simulink model "ClosedLoop_sim"  (Simulink 9.2)
settings: Solver=VariableStepAuto  StartTime=0.0  StopTime=10.0  RelTol=1e-3
libraries: neural x305, simulink x1
(part 1 of 13)
settings Model: Creator=manzand  LastModifiedBy=manzand
settings DataIOCC: LimitDataPoints=off  SaveFormat=Dataset  SignalLoggingSaveFormat=Dataset
settings OptimizationCC: LifeSpan=auto
settings DebuggingCC: UnderspecifiedInitializationDetection=Simplified  MergeDetectMultiDrivingBlocksExec=error  FcnCallInpInsideContextMsg=error  StateNameClashWarn=none  SFUnexpectedBacktrackingDiag=error  SFNoUnconditionalDefaultTransitionDiag=error  SFExecutionAtInitializationDiag=warning
settings HardwareCC: ProdBitPerPointer=64  ProdBitPerSizeT=64  ProdBitPerPtrDiffT=64  ProdLargestAtomicFloat=Float  ProdIntDivRoundTo=Zero  ProdEndianess=LittleEndian  ProdWordSize=64  ProdHWDeviceType=Intel->x86-64 (Windows64)
settings ModelReferenceCC: PropagateSignalLabelsOutOfModel=on
settings SFSimCC: SimUseLocalCustomCode=on
settings RTWCC: RTWUseLocalCustomCode=on
settings CodeAppCC: StateflowObjectComments=off
settings GRTTargetCC: TargetLangStandard=C99 (ISO)  GeneratePreprocessorConditionals=Use local settings  CombineOutputUpdateFcns=on  GRTInterface=off
settings ConfigComp: CovMetricSettings=dwe  CovHtmlReporting=off  CovSaveCumulativeToWorkspaceVar=off  CovSaveSingleToWorkspaceVar=off  CovExternalEMLEnable=on

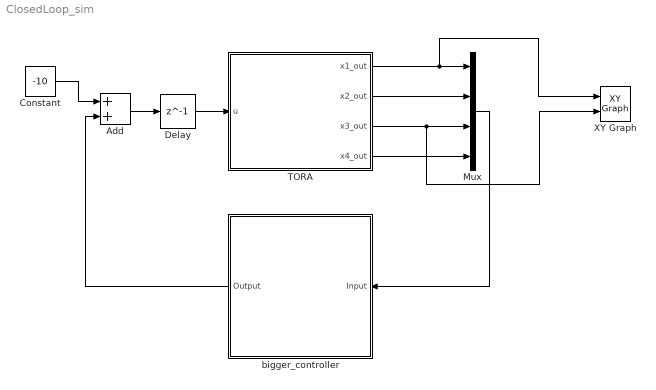
== system ClosedLoop_sim ==
  Add : Sum
  Constant : Constant  Value=-10
  Delay : Delay  DelayLength=1  InitialCondition=0
  Mux : Mux
  TORA : Stateflow chart  TreatAsAtomicUnit=on
  XY Graph : simulink/Sinks/XY Graph  xmin=-1  xmax=1  ymin=-1  ymax=1  st=-1
  bigger_controller : Subsystem
      mask help: Feed-Forward Neural Network
      mask Display: e = 0.06;c1 = [120 150 230]/255;c2 = ([120 150 230]+0)/383;c3 = ([120 150 230]+128)/383;patch([0 1 1 0],[0 0 1 1],c1);patch([0 1 1 1-e 1-e 0+e],[0 0 1 1-e 0+e 0+e],c2);patch([0 0 1 1-e 0+e 0+e],[0 1 1 1-e 1-e 0+e],c3);plot([0 1 1 0 0],[0 0 1 1 0]);fprintf('NNET');port_label('input',1,' Input');port_label('output',1,'Output ');
  wires:
  TORA/1(x1_out) -> XY Graph/1, Mux/1
  TORA/2(x2_out) -> Mux/2
  TORA/3(x3_out) -> XY Graph/2, Mux/3
  TORA/4(x4_out) -> Mux/4
  Add/1 -> Delay/1
  Constant/1 -> Add/1
  Mux/1 -> bigger_controller/1(Input)
  bigger_controller/1(Output) -> Add/2
  Delay/1 -> TORA/1(u)

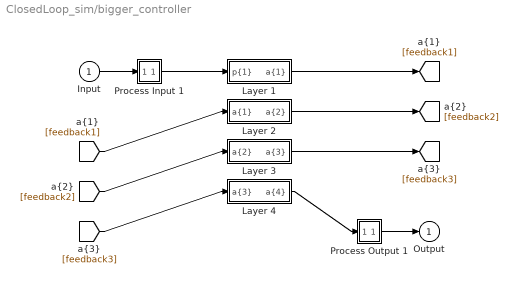
== system ClosedLoop_sim/bigger_controller ==
  Input : Inport  PortDimensions=4
      mask Display: e = 0.06;c1 = [120 230 180]/255;c2 = ([120 230 180]+0)/(256+128);c3 = ([120 230 180]+128)/(256+128);patch([0 1 1 0],[0 0 1 1],c1);patch([0 1 1 1-e 1-e 0+e],[0 0 1 1-e 0+e 0+e],c2);patch([0 0 1 1-e 0+e 0+e],[0 1 1 1-e 1-e 0+e],c3);plot([0 1 1 0 0],[0 0 1 1 0]);
  Layer 1 : Subsystem
      mask Display: e = 0.06;c1 = [120 150 230]/255;c2 = ([120 150 230]+0)/383;c3 = ([120 150 230]+128)/383;patch([0 1 1 0],[0 0 1 1],c1);patch([0 1 1 1-e 1-e 0+e],[0 0 1 1-e 0+e 0+e],c2);patch([0 0 1 1-e 0+e 0+e],[0 1 1 1-e 1-e 0+e],c3);plot([0 1 1 0 0],[0 0 1 1 0]);
  Layer 2 : Subsystem
      mask Display: e = 0.06;c1 = [120 150 230]/255;c2 = ([120 150 230]+0)/383;c3 = ([120 150 230]+128)/383;patch([0 1 1 0],[0 0 1 1],c1);patch([0 1 1 1-e 1-e 0+e],[0 0 1 1-e 0+e 0+e],c2);patch([0 0 1 1-e 0+e 0+e],[0 1 1 1-e 1-e 0+e],c3);plot([0 1 1 0 0],[0 0 1 1 0]);
  Layer 3 : Subsystem
      mask Display: e = 0.06;c1 = [120 150 230]/255;c2 = ([120 150 230]+0)/383;c3 = ([120 150 230]+128)/383;patch([0 1 1 0],[0 0 1 1],c1);patch([0 1 1 1-e 1-e 0+e],[0 0 1 1-e 0+e 0+e],c2);patch([0 0 1 1-e 0+e 0+e],[0 1 1 1-e 1-e 0+e],c3);plot([0 1 1 0 0],[0 0 1 1 0]);
  Layer 4 : Subsystem
      mask Display: e = 0.06;c1 = [120 150 230]/255;c2 = ([120 150 230]+0)/383;c3 = ([120 150 230]+128)/383;patch([0 1 1 0],[0 0 1 1],c1);patch([0 1 1 1-e 1-e 0+e],[0 0 1 1-e 0+e 0+e],c2);patch([0 0 1 1-e 0+e 0+e],[0 1 1 1-e 1-e 0+e],c3);plot([0 1 1 0 0],[0 0 1 1 0]);
  Process Input 1 : Subsystem
      mask Display: e = 0.06;c1 = [120 150 230]/255;c2 = ([120 150 230]+0)/383;c3 = ([120 150 230]+128)/383;patch([0 1 1 0],[0 0 1 1],c1);patch([0 1 1 1-e 1-e 0+e],[0 0 1 1-e 0+e 0+e],c2);patch([0 0 1 1-e 0+e 0+e],[0 1 1 1-e 1-e 0+e],c3);plot([0 1 1 0 0],[0 0 1 1 0]);
  Process Output 1 : Subsystem
      mask Display: e = 0.06;c1 = [120 150 230]/255;c2 = ([120 150 230]+0)/383;c3 = ([120 150 230]+128)/383;patch([0 1 1 0],[0 0 1 1],c1);patch([0 1 1 1-e 1-e 0+e],[0 0 1 1-e 0+e 0+e],c2);patch([0 0 1 1-e 0+e 0+e],[0 1 1 1-e 1-e 0+e],c3);plot([0 1 1 0 0],[0 0 1 1 0]);
  Output : Outport  InitialOutput=0
      mask Display: e = 0.06;c1 = [120 230 180]/255;c2 = ([120 230 180]+0)/(256+128);c3 = ([120 230 180]+128)/(256+128);patch([0 1 1 0],[0 0 1 1],c1);patch([0 1 1 1-e 1-e 0+e],[0 0 1 1-e 0+e 0+e],c2);patch([0 0 1 1-e 0+e 0+e],[0 1 1 1-e 1-e 0+e],c3);plot([0 1 1 0 0],[0 0 1 1 0]);
  wires:
  Layer 4/1("a{4}") -> Process Output 1/1(a)
  [feedback3] -> Layer 4/1("a{3} ")
  Layer 3/1("a{3}") -> [feedback3]
  [feedback2] -> Layer 3/1("a{2} ")
  Layer 2/1("a{2}") -> [feedback2]
  [feedback1] -> Layer 2/1("a{1} ")
  Layer 1/1("a{1}") -> [feedback1]
  Process Input 1/1(p) -> Layer 1/1("p{1}")
  Process Output 1/1(y) -> Output/1
  Input/1 -> Process Input 1/1(x)

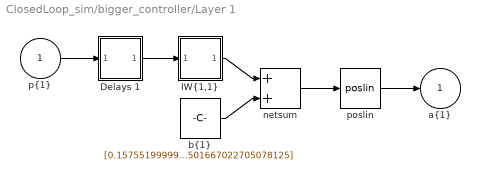
== system ClosedLoop_sim/bigger_controller/Layer 1 ==
  "p{1}" : Inport  PortDimensions=4
      mask Display: e = 0.06;c1 = [120 230 180]/255;c2 = ([120 230 180]+0)/(256+128);c3 = ([120 230 180]+128)/(256+128);patch([0 1 1 0],[0 0 1 1],c1);patch([0 1 1 1-e 1-e 0+e],[0 0 1 1-e 0+e 0+e],c2);patch([0 0 1 1-e 0+e 0+e],[0 1 1 1-e 1-e 0+e],c3);plot([0 1 1 0 0],[0 0 1 1 0]);
  Delays 1 : Subsystem
      mask Display: e = 0.06;c1 = [120 150 230]/255;c2 = ([120 150 230]+0)/383;c3 = ([120 150 230]+128)/383;patch([0 1 1 0],[0 0 1 1],c1);patch([0 1 1 1-e 1-e 0+e],[0 0 1 1-e 0+e 0+e],c2);patch([0 0 1 1-e 0+e 0+e],[0 1 1 1-e 1-e 0+e],c3);plot([0 1 1 0 0],[0 0 1 1 0]);disp('0');
  "IW{1,1}" : Subsystem
      mask Display: e = 0.06;c1 = [120 150 230]/255;c2 = ([120 150 230]+0)/383;c3 = ([120 150 230]+128)/383;patch([0 1 1 0],[0 0 1 1],c1);patch([0 1 1 1-e 1-e 0+e],[0 0 1 1-e 0+e 0+e],c2);patch([0 0 1 1-e 0+e 0+e],[0 1 1 1-e 1-e 0+e],c3);plot([0 1 1 0 0],[0 0 1 1 0]);disp('W');
  "b{1}" : Constant  Value=[0.1575519999999999976036946236490621231496334075927734375;0.17304500000000000436983782492461614310741424560546875;0.2687180000000000124060761663713492453098297119140625;0.179725999999999996870059248976758681237697601318359375;0.040231999999999996930899470726217259652912616729736328125;0.156368000000000006988187806200585328042507171630859375;0.31267699999999998272670609367196448147296905517578125;0.2392579999999999984527931928823818452656269073486328125;0.1582800000000000040234482412415673024952411651611328125;0.2311739999999999906066250332514755427837371826171875;0.2380319999999999935891281666044960729777812957763671875;0.246018999999999987693399816635064780712127685546875;0.236512000000000000010658141036401502788066864013671875;0.2016340000000000076685324756908812560141086578369140625;0.209523999999999988030907616121112369000911712646484375;0.299843000000000026172841671723290346562862396240234375;0.130168000000000005922373702560435049235820770263671875;0.1506659999999999943742778896194067783653736114501953125;0.1991340000000000054480864264405681751668453216552734375;0.189705000000000012505552149377763271331787109375;0.2312309999999999921005411351870861835777759552001953125;0.2230020000000000057749360848902142606675624847412109375;0.23258400000000001295319407290662638843059539794921875;0.107484999999999997211119762141606770455837249755859375;0.253188000000000024147794874807004816830158233642578125;0.20484700000000000130739863379858434200286865234375;0.2490779999999999938520289788357331417500972747802734375;0.32403199999999998670574541392852552235126495361328125;0.1958930000000000115623066676562302745878696441650390625;0.30651200000000000667199628878734074532985687255859375;0.1592550000000000076649797620120807550847530364990234375;0.20692399999999999682387397115235216915607452392578125;0.1734940000000000093205443363331141881644725799560546875;0.2635899999999999909761072558467276394367218017578125;0.201423999999999991938892662801663391292095184326171875;0.2122179999999999899795710689431871287524700164794921875;0.062077000000000000234923192010683123953640460968017578125;0.1976620000000000043627323975670151412487030029296875;0.10692300000000000415045775525868521071970462799072265625;0.22057599999999999429434183184639550745487213134765625;0.211060999999999998610888951589004136621952056884765625;0.165831000000000006178169087434071116149425506591796875;0.2300419999999999964845898148269043304026126861572265625;0.2126230000000000064375171859865076839923858642578125;0.22377700000000000368771679859491996467113494873046875;0.2484480000000000021742607714259065687656402587890625;0.1790090000000000014512835377900046296417713165283203125;0.300943000000000016047607687141862697899341583251953125;0.22207399999999999362643166023190133273601531982421875;0.1654730000000000089688256821318645961582660675048828125;0.3032880000000000020321522242738865315914154052734375;0.1556530000000000135695898961785132996737957000732421875;0.1670599999999999862865251998300664126873016357421875;0.227673999999999987498000564301037229597568511962890625;0.176128000000000006775024985472555272281169891357421875;0.2231769999999999865014643773974967189133167266845703125;0.279793000000000013915979479861562140285968780517578125;0.23367999999999999882760448599583469331264495849609375;0.164144000000000012118306358388508670032024383544921875;0.228663000000000005140776693224324844777584075927734375;0.1560140000000000137792000032277428545057773590087890625;0.195535999999999987597476547307451255619525909423828125;0.1807410000000000127595711774119990877807140350341796875;0.16601399999999999490540858460008166730403900146484375;0.1955820000000000058459903584662242792546749114990234375;0.206423999999999996379784761302289552986621856689453125;0.15153600000000000402877731175976805388927459716796875;0.325442999999999982296827738537103869020938873291015625;0.1548029999999999961612928700560587458312511444091796875;0.252504000000000006220801651579677127301692962646484375 ...(+1711 chars)]
      mask Display: e = 0.06;c1 = [120 150 230]/255;c2 = ([120 150 230]+0)/383;c3 = ([120 150 230]+128)/383;patch([0 1 1 0],[0 0 1 1],c1);patch([0 1 1 1-e 1-e 0+e],[0 0 1 1-e 0+e 0+e],c2);patch([0 0 1 1-e 0+e 0+e],[0 1 1 1-e 1-e 0+e],c3);plot([0 1 1 0 0],[0 0 1 1 0]);disp('b');
  netsum : Sum  Inputs=2  SaturateOnIntegerOverflow=on  InputSameDT=on  OutDataTypeStr=Inherit: Same as first input
      mask Display: e = 0.06;c1 = [120 150 230]/255;c2 = ([120 150 230]+0)/383;c3 = ([120 150 230]+128)/383;patch([0 1 1 0],[0 0 1 1],c1);patch([0 1 1 1-e 1-e 0+e],[0 0 1 1-e 0+e 0+e],c2);patch([0 0 1 1-e 0+e 0+e],[0 1 1 1-e 1-e 0+e],c3);plot([0 1 1 0 0],[0 0 1 1 0]);disp('+');
  poslin : neural/Transfer Functions/poslin
      settings: SourceProductName=Neural Network Toolbox  SourceProductBaseCode=NN
  "a{1}" : Outport  InitialOutput=[0;0;0;0;0;0;0;0;0;0;0;0;0;0;0;0;0;0;0;0;0;0;0;0;0;0;0;0;0;0;0;0;0;0;0;0;0;0;0;0;0;0;0;0;0;0;0;0;0;0;0;0;0;0;0;0;0;0;0;0;0;0;0;0;0;0;0;0;0;0;0;0;0;0;0;0;0;0;0;0;0;0;0;0;0;0;0;0;0;0;0;0;0;0;0;0;0;0;0;0]
      mask Display: e = 0.06;c1 = [120 230 180]/255;c2 = ([120 230 180]+0)/(256+128);c3 = ([120 230 180]+128)/(256+128);patch([0 1 1 0],[0 0 1 1],c1);patch([0 1 1 1-e 1-e 0+e],[0 0 1 1-e 0+e 0+e],c2);patch([0 0 1 1-e 0+e 0+e],[0 1 1 1-e 1-e 0+e],c3);plot([0 1 1 0 0],[0 0 1 1 0]);
  wires:
  poslin/1 -> "a{1}"/1
  netsum/1 -> poslin/1
  "b{1}"/1 -> netsum/2
  "IW{1,1}"/1("iz{1,1}") -> netsum/1
  Delays 1/1("pd{1,1}") -> "IW{1,1}"/1("pd{1,1}")
  "p{1}"/1 -> Delays 1/1("p{1}")

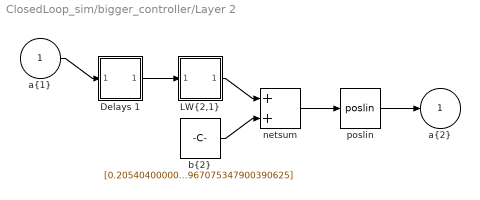
== system ClosedLoop_sim/bigger_controller/Layer 2 ==
  "a{1} " : Inport  PortDimensions=100
      mask Display: e = 0.06;c1 = [120 230 180]/255;c2 = ([120 230 180]+0)/(256+128);c3 = ([120 230 180]+128)/(256+128);patch([0 1 1 0],[0 0 1 1],c1);patch([0 1 1 1-e 1-e 0+e],[0 0 1 1-e 0+e 0+e],c2);patch([0 0 1 1-e 0+e 0+e],[0 1 1 1-e 1-e 0+e],c3);plot([0 1 1 0 0],[0 0 1 1 0]);
  Delays 1 : Subsystem
      mask Display: e = 0.06;c1 = [120 150 230]/255;c2 = ([120 150 230]+0)/383;c3 = ([120 150 230]+128)/383;patch([0 1 1 0],[0 0 1 1],c1);patch([0 1 1 1-e 1-e 0+e],[0 0 1 1-e 0+e 0+e],c2);patch([0 0 1 1-e 0+e 0+e],[0 1 1 1-e 1-e 0+e],c3);plot([0 1 1 0 0],[0 0 1 1 0]);disp('0');
  "LW{2,1}" : Subsystem
      mask Display: e = 0.06;c1 = [120 150 230]/255;c2 = ([120 150 230]+0)/383;c3 = ([120 150 230]+128)/383;patch([0 1 1 0],[0 0 1 1],c1);patch([0 1 1 1-e 1-e 0+e],[0 0 1 1-e 0+e 0+e],c2);patch([0 0 1 1-e 0+e 0+e],[0 1 1 1-e 1-e 0+e],c3);plot([0 1 1 0 0],[0 0 1 1 0]);disp('W');
  "b{2}" : Constant  Value=[0.2054040000000000032454039455842575989663600921630859375;0.24318600000000001326583287664107047021389007568359375;0.16940399999999999902655645200866274535655975341796875;0.1861800000000000121502807814977131783962249755859375;0.2091220000000000023288038164537283591926097869873046875;0.1638300000000000034017233474514796398580074310302734375;0.163463999999999998191668737490545026957988739013671875;0.1972500000000000086597395920762210153043270111083984375;0.2316930000000000100524033541660173796117305755615234375;0.206347000000000002639666263348772190511226654052734375;0.2179270000000000095941032896007527597248554229736328125;0.289185999999999998610888951589004136621952056884765625;0.23429800000000000625988150204648263752460479736328125;0.285609999999999975006659269638475961983203887939453125;0.300897000000000025554669491612003184854984283447265625;0.25646299999999999652544602213311009109020233154296875;0.181130999999999986460608170091290958225727081298828125;0.14595700000000000340349970429087989032268524169921875;0.1714350000000000040500935938325710594654083251953125;0.21252999999999999669597627871553413569927215576171875;0.29249000000000002774669383143191225826740264892578125;0.08343299999999999327915389812915236689150333404541015625;0.19251099999999998768629438927746377885341644287109375;0.166696000000000010832224006662727333605289459228515625;0.2175920000000000076312289820634759962558746337890625;0.318350999999999995093702409576508216559886932373046875;0.1235020000000000006679101716144941747188568115234375;0.2268860000000000043396397586548118852078914642333984375;0.2413849999999999884625623280953732319176197052001953125;0.2428329999999999933013583586216554976999759674072265625;0.191359000000000001318056774834985844790935516357421875;0.295406000000000001914912672873470000922679901123046875;0.149309999999999998276933865781757049262523651123046875;0.1480889999999999984137133424155763350427150726318359375;0.2849369999999999958362195684458129107952117919921875;0.2124769999999999992024157791092875413596630096435546875;0.1831170000000000019912960169676807709038257598876953125;0.297933000000000003382183422218076884746551513671875;0.2229669999999999985274001801371923647820949554443359375;0.122661999999999993260502151315449737012386322021484375;0.1719400000000000094946273065943387337028980255126953125;0.2316499999999999948041562447542673908174037933349609375;0.10961300000000000209876560575139592401683330535888671875;0.289393999999999984584775347684626467525959014892578125;0.15987899999999999334221456592786125838756561279296875;0.279397999999999979703346753012738190591335296630859375;0.1705379999999999951487694715979159809648990631103515625;0.131487999999999993772092921062721870839595794677734375;0.1853269999999999917417170536282355897128582000732421875;0.1466139999999999943280926117950002662837505340576171875;0.1771649999999999891553414954614709131419658660888671875;0.315174999999999982946974341757595539093017578125;0.185771999999999992692067962707369588315486907958984375;0.170611000000000012644107982850982807576656341552734375;0.2083790000000000086632923057550215162336826324462890625;0.2174460000000000003961275751862558536231517791748046875;0.16120000000000000994759830064140260219573974609375;0.1419499999999999928501637214139918796718120574951171875;0.1647800000000000097966079692923813126981258392333984375;0.201440000000000007940315072119119577109813690185546875;0.2291009999999999990905052982270717620849609375;0.2059580000000000021831425556229078210890293121337890625;0.08723300000000000498090457767830230295658111572265625;0.1885940000000000116298082275534397922456264495849609375;0.1459910000000000096509467084615607745945453643798828125;0.0826240000000000029967139880682225339114665985107421875;0.10283299999999999385646987093423376791179180145263671875;0.256008000000000013329781722859479486942291259765625;0.198189000000000004053646307511371560394763946533203125;0.11502700000000000424282831090749823488295078277587890625 ...(+1711 chars)]
      mask Display: e = 0.06;c1 = [120 150 230]/255;c2 = ([120 150 230]+0)/383;c3 = ([120 150 230]+128)/383;patch([0 1 1 0],[0 0 1 1],c1);patch([0 1 1 1-e 1-e 0+e],[0 0 1 1-e 0+e 0+e],c2);patch([0 0 1 1-e 0+e 0+e],[0 1 1 1-e 1-e 0+e],c3);plot([0 1 1 0 0],[0 0 1 1 0]);disp('b');
  netsum : Sum  Inputs=2  SaturateOnIntegerOverflow=on  InputSameDT=on  OutDataTypeStr=Inherit: Same as first input
      mask Display: e = 0.06;c1 = [120 150 230]/255;c2 = ([120 150 230]+0)/383;c3 = ([120 150 230]+128)/383;patch([0 1 1 0],[0 0 1 1],c1);patch([0 1 1 1-e 1-e 0+e],[0 0 1 1-e 0+e 0+e],c2);patch([0 0 1 1-e 0+e 0+e],[0 1 1 1-e 1-e 0+e],c3);plot([0 1 1 0 0],[0 0 1 1 0]);disp('+');
  poslin : neural/Transfer Functions/poslin
      settings: SourceProductName=Neural Network Toolbox  SourceProductBaseCode=NN
  "a{2}" : Outport  InitialOutput=[0;0;0;0;0;0;0;0;0;0;0;0;0;0;0;0;0;0;0;0;0;0;0;0;0;0;0;0;0;0;0;0;0;0;0;0;0;0;0;0;0;0;0;0;0;0;0;0;0;0;0;0;0;0;0;0;0;0;0;0;0;0;0;0;0;0;0;0;0;0;0;0;0;0;0;0;0;0;0;0;0;0;0;0;0;0;0;0;0;0;0;0;0;0;0;0;0;0;0;0]
      mask Display: e = 0.06;c1 = [120 230 180]/255;c2 = ([120 230 180]+0)/(256+128);c3 = ([120 230 180]+128)/(256+128);patch([0 1 1 0],[0 0 1 1],c1);patch([0 1 1 1-e 1-e 0+e],[0 0 1 1-e 0+e 0+e],c2);patch([0 0 1 1-e 0+e 0+e],[0 1 1 1-e 1-e 0+e],c3);plot([0 1 1 0 0],[0 0 1 1 0]);
  wires:
  poslin/1 -> "a{2}"/1
  netsum/1 -> poslin/1
  "b{2}"/1 -> netsum/2
  "LW{2,1}"/1("lz{2,1}") -> netsum/1
  Delays 1/1("pd{2,1}") -> "LW{2,1}"/1("ad{2,1}")
  "a{1} "/1 -> Delays 1/1("p{2}")

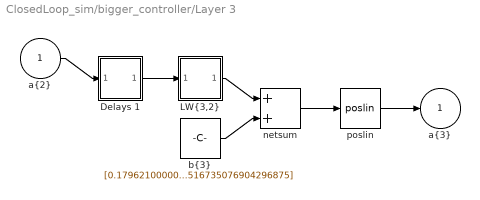
== system ClosedLoop_sim/bigger_controller/Layer 3 ==
  "a{2} " : Inport  PortDimensions=100
      mask Display: e = 0.06;c1 = [120 230 180]/255;c2 = ([120 230 180]+0)/(256+128);c3 = ([120 230 180]+128)/(256+128);patch([0 1 1 0],[0 0 1 1],c1);patch([0 1 1 1-e 1-e 0+e],[0 0 1 1-e 0+e 0+e],c2);patch([0 0 1 1-e 0+e 0+e],[0 1 1 1-e 1-e 0+e],c3);plot([0 1 1 0 0],[0 0 1 1 0]);
  Delays 1 : Subsystem
      mask Display: e = 0.06;c1 = [120 150 230]/255;c2 = ([120 150 230]+0)/383;c3 = ([120 150 230]+128)/383;patch([0 1 1 0],[0 0 1 1],c1);patch([0 1 1 1-e 1-e 0+e],[0 0 1 1-e 0+e 0+e],c2);patch([0 0 1 1-e 0+e 0+e],[0 1 1 1-e 1-e 0+e],c3);plot([0 1 1 0 0],[0 0 1 1 0]);disp('0');
  "LW{3,2}" : Subsystem
      mask Display: e = 0.06;c1 = [120 150 230]/255;c2 = ([120 150 230]+0)/383;c3 = ([120 150 230]+128)/383;patch([0 1 1 0],[0 0 1 1],c1);patch([0 1 1 1-e 1-e 0+e],[0 0 1 1-e 0+e 0+e],c2);patch([0 0 1 1-e 0+e 0+e],[0 1 1 1-e 1-e 0+e],c3);plot([0 1 1 0 0],[0 0 1 1 0]);disp('W');
  "b{3}" : Constant  Value=[0.1796210000000000028830271503466065041720867156982421875;0.1377839999999999898161462397183640860021114349365234375;0.2014869999999999994333421682313201017677783966064453125;0.1803450000000000053024251656097476370632648468017578125;0.20910200000000001008260142043582163751125335693359375;0.1752180000000000126281207712963805533945560455322265625;0.2049789999999999945412554325230303220450878143310546875;0.13145200000000001328004373135627247393131256103515625;0.1911170000000000090967233745686826296150684356689453125;0.2256479999999999874749079253888339735567569732666015625;0.197778000000000009350742402602918446063995361328125;0.1411320000000000074447115139264496974647045135498046875;0.264944000000000012828849094148608855903148651123046875;0.2711580000000000101323394119390286505222320556640625;0.258637999999999979028331154040643014013767242431640625;0.273583999999999993857358049353933893144130706787109375;0.24693799999999999084110413605230860412120819091796875;0.11205800000000000482547335423078038729727268218994140625;0.260473000000000010079048706757021136581897735595703125;0.273475999999999996870059248976758681237697601318359375;0.2004410000000000080522255530013353563845157623291015625;0.29754199999999997316990629769861698150634765625;0.1733820000000000083328899336265749298036098480224609375;0.154911999999999994148680571015574969351291656494140625;0.233968000000000009297451697420910932123661041259765625;0.2221499999999999863664612576030776835978031158447265625;0.1614960000000000006625811010962934233248233795166015625;0.210235000000000005204725539442733861505985260009765625;0.1426800000000000012700951401711790822446346282958984375;0.147000999999999992784438518356182612478733062744140625;0.1915050000000000085531581817122059874236583709716796875;0.2057350000000000012079226507921703159809112548828125;0.179896000000000000351718654201249592006206512451171875;0.1480700000000000071675998469800106249749660491943359375;0.12618899999999999561595132036018185317516326904296875;0.143332999999999988194332445345935411751270294189453125;0.239095000000000001971756091734278015792369842529296875;0.246356999999999992656540825919364579021930694580078125;0.244993999999999989558574498005327768623828887939453125;0.1976650000000000073629990993140381760895252227783203125;0.1484600000000000086242124552882160060107707977294921875;0.2175539999999999973834263755634310655295848846435546875;0.2183549999999999935429428887800895608961582183837890625;0.2311999999999999888533608327634283341467380523681640625;0.2306080000000000074233952318536466918885707855224609375;0.2131039999999999878799172847720910795032978057861328125;0.19639200000000001100630697692395187914371490478515625;0.180539000000000005030642569181509315967559814453125;0.2338590000000000113100639964613947086036205291748046875;0.25612299999999998956212721168412826955318450927734375;0.254707999999999989970689284746185876429080963134765625;0.2510419999999999873807610129006206989288330078125;0.274374999999999980015985556747182272374629974365234375;0.1979849999999999943245398981161997653543949127197265625;0.187753000000000003222311306672054342925548553466796875;0.1910789999999999988489207680686376988887786865234375;0.1640149999999999941291406457821722142398357391357421875;0.2096099999999999907718262193156988359987735748291015625;0.2399630000000000096260777127099572680890560150146484375;0.1912480000000000013304912727107875980436801910400390625;0.2447719999999999895834434937569312751293182373046875;0.2153869999999999951256768326857127249240875244140625;0.2286390000000000088942186948770540766417980194091796875;0.153812000000000004273914555597002618014812469482421875;0.17943100000000000715516534910420887172222137451171875;0.11904900000000000204192218689058790914714336395263671875;0.256979000000000012970957641300628893077373504638671875;0.112287999999999998923527755323448218405246734619140625;0.2147489999999999954471974206171580590307712554931640625;0.24546699999999999075583900776109658181667327880859375 ...(+1695 chars)]
      mask Display: e = 0.06;c1 = [120 150 230]/255;c2 = ([120 150 230]+0)/383;c3 = ([120 150 230]+128)/383;patch([0 1 1 0],[0 0 1 1],c1);patch([0 1 1 1-e 1-e 0+e],[0 0 1 1-e 0+e 0+e],c2);patch([0 0 1 1-e 0+e 0+e],[0 1 1 1-e 1-e 0+e],c3);plot([0 1 1 0 0],[0 0 1 1 0]);disp('b');
  netsum : Sum  Inputs=2  SaturateOnIntegerOverflow=on  InputSameDT=on  OutDataTypeStr=Inherit: Same as first input
      mask Display: e = 0.06;c1 = [120 150 230]/255;c2 = ([120 150 230]+0)/383;c3 = ([120 150 230]+128)/383;patch([0 1 1 0],[0 0 1 1],c1);patch([0 1 1 1-e 1-e 0+e],[0 0 1 1-e 0+e 0+e],c2);patch([0 0 1 1-e 0+e 0+e],[0 1 1 1-e 1-e 0+e],c3);plot([0 1 1 0 0],[0 0 1 1 0]);disp('+');
  poslin : neural/Transfer Functions/poslin
      settings: SourceProductName=Neural Network Toolbox  SourceProductBaseCode=NN
  "a{3}" : Outport  InitialOutput=[0;0;0;0;0;0;0;0;0;0;0;0;0;0;0;0;0;0;0;0;0;0;0;0;0;0;0;0;0;0;0;0;0;0;0;0;0;0;0;0;0;0;0;0;0;0;0;0;0;0;0;0;0;0;0;0;0;0;0;0;0;0;0;0;0;0;0;0;0;0;0;0;0;0;0;0;0;0;0;0;0;0;0;0;0;0;0;0;0;0;0;0;0;0;0;0;0;0;0;0]
      mask Display: e = 0.06;c1 = [120 230 180]/255;c2 = ([120 230 180]+0)/(256+128);c3 = ([120 230 180]+128)/(256+128);patch([0 1 1 0],[0 0 1 1],c1);patch([0 1 1 1-e 1-e 0+e],[0 0 1 1-e 0+e 0+e],c2);patch([0 0 1 1-e 0+e 0+e],[0 1 1 1-e 1-e 0+e],c3);plot([0 1 1 0 0],[0 0 1 1 0]);
  wires:
  poslin/1 -> "a{3}"/1
  netsum/1 -> poslin/1
  "b{3}"/1 -> netsum/2
  "LW{3,2}"/1("lz{3,2}") -> netsum/1
  Delays 1/1("pd{3,2}") -> "LW{3,2}"/1("ad{3,2}")
  "a{2} "/1 -> Delays 1/1("p{3}")

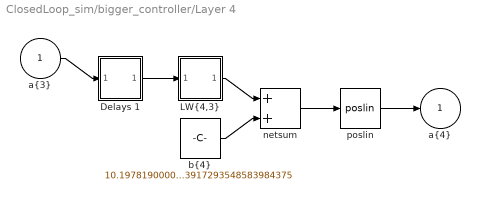
== system ClosedLoop_sim/bigger_controller/Layer 4 ==
  "a{3} " : Inport  PortDimensions=100
      mask Display: e = 0.06;c1 = [120 230 180]/255;c2 = ([120 230 180]+0)/(256+128);c3 = ([120 230 180]+128)/(256+128);patch([0 1 1 0],[0 0 1 1],c1);patch([0 1 1 1-e 1-e 0+e],[0 0 1 1-e 0+e 0+e],c2);patch([0 0 1 1-e 0+e 0+e],[0 1 1 1-e 1-e 0+e],c3);plot([0 1 1 0 0],[0 0 1 1 0]);
  Delays 1 : Subsystem
      mask Display: e = 0.06;c1 = [120 150 230]/255;c2 = ([120 150 230]+0)/383;c3 = ([120 150 230]+128)/383;patch([0 1 1 0],[0 0 1 1],c1);patch([0 1 1 1-e 1-e 0+e],[0 0 1 1-e 0+e 0+e],c2);patch([0 0 1 1-e 0+e 0+e],[0 1 1 1-e 1-e 0+e],c3);plot([0 1 1 0 0],[0 0 1 1 0]);disp('0');
  "LW{4,3}" : Subsystem
      mask Display: e = 0.06;c1 = [120 150 230]/255;c2 = ([120 150 230]+0)/383;c3 = ([120 150 230]+128)/383;patch([0 1 1 0],[0 0 1 1],c1);patch([0 1 1 1-e 1-e 0+e],[0 0 1 1-e 0+e 0+e],c2);patch([0 0 1 1-e 0+e 0+e],[0 1 1 1-e 1-e 0+e],c3);plot([0 1 1 0 0],[0 0 1 1 0]);disp('W');
  "b{4}" : Constant  Value=10.1978190000000008552660801797173917293548583984375
      mask Display: e = 0.06;c1 = [120 150 230]/255;c2 = ([120 150 230]+0)/383;c3 = ([120 150 230]+128)/383;patch([0 1 1 0],[0 0 1 1],c1);patch([0 1 1 1-e 1-e 0+e],[0 0 1 1-e 0+e 0+e],c2);patch([0 0 1 1-e 0+e 0+e],[0 1 1 1-e 1-e 0+e],c3);plot([0 1 1 0 0],[0 0 1 1 0]);disp('b');
  netsum : Sum  Inputs=2  SaturateOnIntegerOverflow=on  InputSameDT=on  OutDataTypeStr=Inherit: Same as first input
      mask Display: e = 0.06;c1 = [120 150 230]/255;c2 = ([120 150 230]+0)/383;c3 = ([120 150 230]+128)/383;patch([0 1 1 0],[0 0 1 1],c1);patch([0 1 1 1-e 1-e 0+e],[0 0 1 1-e 0+e 0+e],c2);patch([0 0 1 1-e 0+e 0+e],[0 1 1 1-e 1-e 0+e],c3);plot([0 1 1 0 0],[0 0 1 1 0]);disp('+');
  poslin : neural/Transfer Functions/poslin
      settings: SourceProductName=Neural Network Toolbox  SourceProductBaseCode=NN
  "a{4}" : Outport  InitialOutput=0
      mask Display: e = 0.06;c1 = [120 230 180]/255;c2 = ([120 230 180]+0)/(256+128);c3 = ([120 230 180]+128)/(256+128);patch([0 1 1 0],[0 0 1 1],c1);patch([0 1 1 1-e 1-e 0+e],[0 0 1 1-e 0+e 0+e],c2);patch([0 0 1 1-e 0+e 0+e],[0 1 1 1-e 1-e 0+e],c3);plot([0 1 1 0 0],[0 0 1 1 0]);
  wires:
  poslin/1 -> "a{4}"/1
  netsum/1 -> poslin/1
  "b{4}"/1 -> netsum/2
  "LW{4,3}"/1("lz{4,3}") -> netsum/1
  Delays 1/1("pd{4,3}") -> "LW{4,3}"/1("ad{4,3}")
  "a{3} "/1 -> Delays 1/1("p{4}")

== system ClosedLoop_sim/bigger_controller/Process Input 1 ==
  x : Inport  PortDimensions=4
      mask Display: e = 0.06;c1 = [120 230 180]/255;c2 = ([120 230 180]+0)/(256+128);c3 = ([120 230 180]+128)/(256+128);patch([0 1 1 0],[0 0 1 1],c1);patch([0 1 1 1-e 1-e 0+e],[0 0 1 1-e 0+e 0+e],c2);patch([0 0 1 1-e 0+e 0+e],[0 1 1 1-e 1-e 0+e],c3);plot([0 1 1 0 0],[0 0 1 1 0]);
  p : Outport  PortDimensions=4
      mask Display: e = 0.06;c1 = [120 230 180]/255;c2 = ([120 230 180]+0)/(256+128);c3 = ([120 230 180]+128)/(256+128);patch([0 1 1 0],[0 0 1 1],c1);patch([0 1 1 1-e 1-e 0+e],[0 0 1 1-e 0+e 0+e],c2);patch([0 0 1 1-e 0+e 0+e],[0 1 1 1-e 1-e 0+e],c3);plot([0 1 1 0 0],[0 0 1 1 0]);
  wires:
  x/1 -> p/1

== system ClosedLoop_sim/bigger_controller/Process Output 1 ==
  a : Inport  PortDimensions=1
      mask Display: e = 0.06;c1 = [120 230 180]/255;c2 = ([120 230 180]+0)/(256+128);c3 = ([120 230 180]+128)/(256+128);patch([0 1 1 0],[0 0 1 1],c1);patch([0 1 1 1-e 1-e 0+e],[0 0 1 1-e 0+e 0+e],c2);patch([0 0 1 1-e 0+e 0+e],[0 1 1 1-e 1-e 0+e],c3);plot([0 1 1 0 0],[0 0 1 1 0]);
  y : Outport  PortDimensions=1
      mask Display: e = 0.06;c1 = [120 230 180]/255;c2 = ([120 230 180]+0)/(256+128);c3 = ([120 230 180]+128)/(256+128);patch([0 1 1 0],[0 0 1 1],c1);patch([0 1 1 1-e 1-e 0+e],[0 0 1 1-e 0+e 0+e],c2);patch([0 0 1 1-e 0+e 0+e],[0 1 1 1-e 1-e 0+e],c3);plot([0 1 1 0 0],[0 0 1 1 0]);
  wires:
  a/1 -> y/1

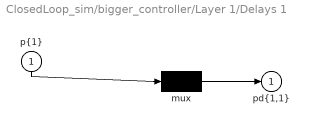
== system ClosedLoop_sim/bigger_controller/Layer 1/Delays 1 ==
  "p{1}" : Inport  PortDimensions=4
      mask Display: e = 0.06;c1 = [120 230 180]/255;c2 = ([120 230 180]+0)/(256+128);c3 = ([120 230 180]+128)/(256+128);patch([0 1 1 0],[0 0 1 1],c1);patch([0 1 1 1-e 1-e 0+e],[0 0 1 1-e 0+e 0+e],c2);patch([0 0 1 1-e 0+e 0+e],[0 1 1 1-e 1-e 0+e],c3);plot([0 1 1 0 0],[0 0 1 1 0]);
  mux : Mux  Inputs=1
      mask Display: e = 0.06;c1 = [120 150 230]/255;c2 = ([120 150 230]+0)/383;c3 = ([120 150 230]+128)/383;patch([0 1 1 0],[0 0 1 1],c1);patch([0 1 1 1-e 1-e 0+e],[0 0 1 1-e 0+e 0+e],c2);patch([0 0 1 1-e 0+e 0+e],[0 1 1 1-e 1-e 0+e],c3);plot([0 1 1 0 0],[0 0 1 1 0]);disp('Mux')
  "pd{1,1}" : Outport
      mask Display: e = 0.06;c1 = [120 230 180]/255;c2 = ([120 230 180]+0)/(256+128);c3 = ([120 230 180]+128)/(256+128);patch([0 1 1 0],[0 0 1 1],c1);patch([0 1 1 1-e 1-e 0+e],[0 0 1 1-e 0+e 0+e],c2);patch([0 0 1 1-e 0+e 0+e],[0 1 1 1-e 1-e 0+e],c3);plot([0 1 1 0 0],[0 0 1 1 0]);
  wires:
  mux/1 -> "pd{1,1}"/1
  "p{1}"/1 -> mux/1
